simulink model "attitudeControllerSim"  (R2015b)
settings: Solver=VariableStepAuto  StartTime=0.0  StopTime=2  RelTol=1e-3
values from neighbouring files (symbols this model uses):
  pitch_ref = 0    [xyzController.m]
  roll_ref = 1    [xyzController.m]
undefined symbols (not defined in the file or in its folder): A12, Fg, Jx, Jy, Jz, kd, kth, L, Lobs, m, w1_bar, w2_bar, w3_bar, w4_bar
settings Model: Creator=USUARIO  LastModifiedBy=USUARIO

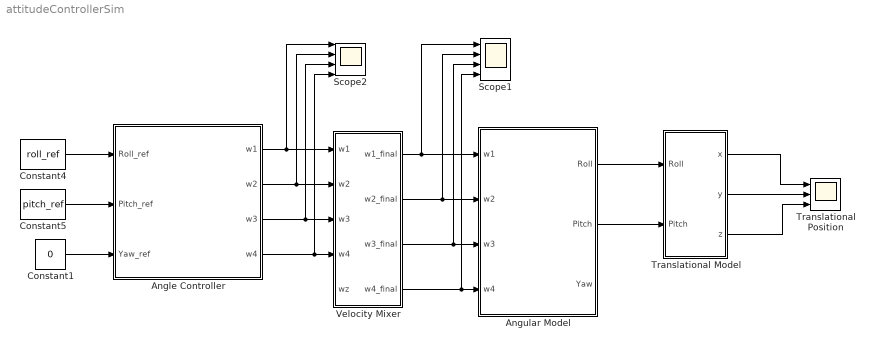
== system attitudeControllerSim ==
  Angle Controller : Subsystem
  Angular Model : Subsystem
  Constant1 : Constant  Value=0
  Constant4 : Constant  Value=roll_ref
  Constant5 : Constant  Value=pitch_ref
  Scope1 : Scope  NumInputPorts=4
  Scope2 : Scope  NumInputPorts=4
  Translational Position : Scope  NumInputPorts=3
  Translational Model : Subsystem
  Velocity Mixer : Subsystem
  wires:
  Constant1/1 -> Angle Controller/3(Yaw_ref)
  Velocity Mixer/1(w1_final) -> Scope1/1, Angular Model/1(w1)
  Velocity Mixer/2(w2_final) -> Scope1/2, Angular Model/2(w2)
  Velocity Mixer/3(w3_final) -> Scope1/3, Angular Model/3(w3)
  Velocity Mixer/4(w4_final) -> Scope1/4, Angular Model/4(w4)
  Angle Controller/1(w1) -> Velocity Mixer/1(w1), Scope2/1
  Angle Controller/2(w2) -> Velocity Mixer/2(w2), Scope2/2
  Angle Controller/3(w3) -> Velocity Mixer/3(w3), Scope2/3
  Angle Controller/4(w4) -> Velocity Mixer/4(w4), Scope2/4
  Angular Model/1(Roll) -> Translational Model/1(Roll)
  Translational Model/1(x) -> Translational Position/1
  Translational Model/2(y) -> Translational Position/2
  Translational Model/3(z) -> Translational Position/3
  Angular Model/2(Pitch) -> Translational Model/2(Pitch)
  Constant4/1 -> Angle Controller/1(Roll_ref)
  Constant5/1 -> Angle Controller/2(Pitch_ref)

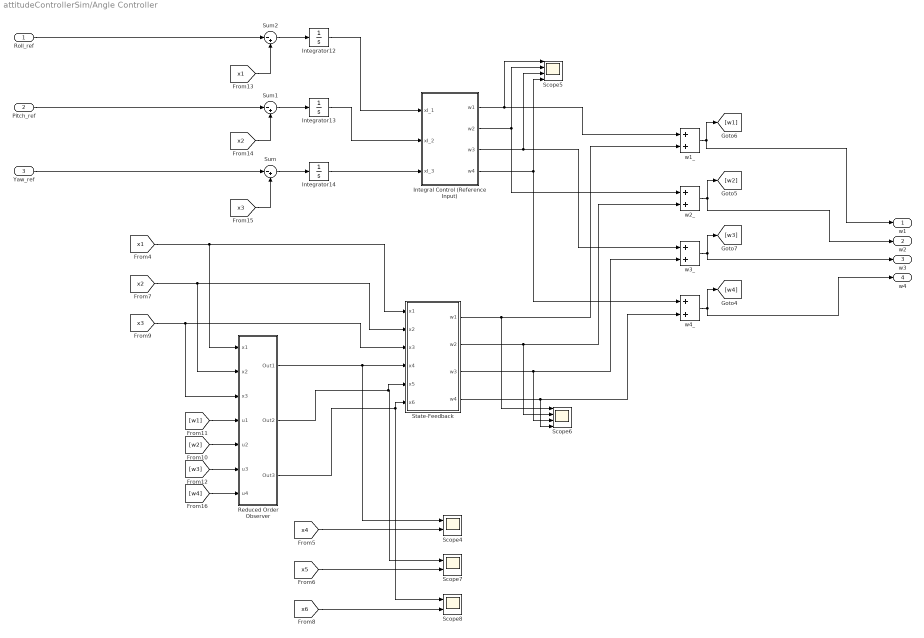
== system attitudeControllerSim/Angle Controller ==
  Roll_ref : Inport
  Pitch_ref : Inport  Port=2
  Yaw_ref : Inport  Port=3
  Integral Control (Reference Input) : MATLAB Function  TreatAsAtomicUnit=on
  Integrator12 : Integrator
  Integrator13 : Integrator
  Integrator14 : Integrator
  Reduced Order Observer : Subsystem
  Scope4 : Scope  NumInputPorts=2
  Scope5 : Scope  NumInputPorts=4
  Scope6 : Scope  NumInputPorts=4
  Scope7 : Scope  NumInputPorts=2
  Scope8 : Scope  NumInputPorts=2
  "State-Feedback " : MATLAB Function  TreatAsAtomicUnit=on
  Sum : Sum  Inputs=|-+
  Sum1 : Sum  Inputs=|-+
  Sum2 : Sum  Inputs=|-+
  w1_ : Sum
  w2_ : Sum
  w3_ : Sum
  w4_ : Sum
  w1 : Outport
  w2 : Outport  Port=2
  w3 : Outport  Port=3
  w4 : Outport  Port=4
  wires:
  "State-Feedback "/4(w4) -> w4_/2, Scope6/4
  Roll_ref/1 -> Sum2/1
  [x3] -> Sum/2
  [x1] -> Sum2/2
  Integrator13/1 -> Integral Control (Reference Input)/2(xI_2)
  "State-Feedback "/1(w1) -> w1_/2, Scope6/1
  [w3] -> Reduced Order Observer/6(u3)
  Sum2/1 -> Integrator12/1
  Sum/1 -> Integrator14/1
  [x3] -> "State-Feedback "/3(x3), Reduced Order Observer/3(x3)
  [w2] -> Reduced Order Observer/5(u2)
  Pitch_ref/1 -> Sum1/1
  Integrator14/1 -> Integral Control (Reference Input)/3(xI_3)
  Reduced Order Observer/3(Out3) -> "State-Feedback "/6(x6), Scope8/1
  [x4] -> Scope4/2
  [x6] -> Scope8/2
  "State-Feedback "/2(w2) -> w2_/2, Scope6/2
  Integral Control (Reference Input)/2(w2) -> Scope5/2, w2_/1
  [w4] -> Reduced Order Observer/7(u4)
  Integral Control (Reference Input)/3(w3) -> w3_/1, Scope5/3
  Reduced Order Observer/2(Out2) -> "State-Feedback "/5(x5), Scope7/1
  [x1] -> "State-Feedback "/1(x1), Reduced Order Observer/1(x1)
  [w1] -> Reduced Order Observer/4(u1)
  Integrator12/1 -> Integral Control (Reference Input)/1(xI_1)
  [x2] -> Sum1/2
  Integral Control (Reference Input)/4(w4) -> Scope5/4, w4_/1
  Integral Control (Reference Input)/1(w1) -> w1_/1, Scope5/1
  [x2] -> "State-Feedback "/2(x2), Reduced Order Observer/2(x2)
  Reduced Order Observer/1(Out1) -> "State-Feedback "/4(x4), Scope4/1
  [x5] -> Scope7/2
  Sum1/1 -> Integrator13/1
  Yaw_ref/1 -> Sum/1
  "State-Feedback "/3(w3) -> w3_/2, Scope6/3
  w1_/1 -> w1/1, [w1]
  w4_/1 -> w4/1, [w4]
  w2_/1 -> w2/1, [w2]
  w3_/1 -> w3/1, [w3]

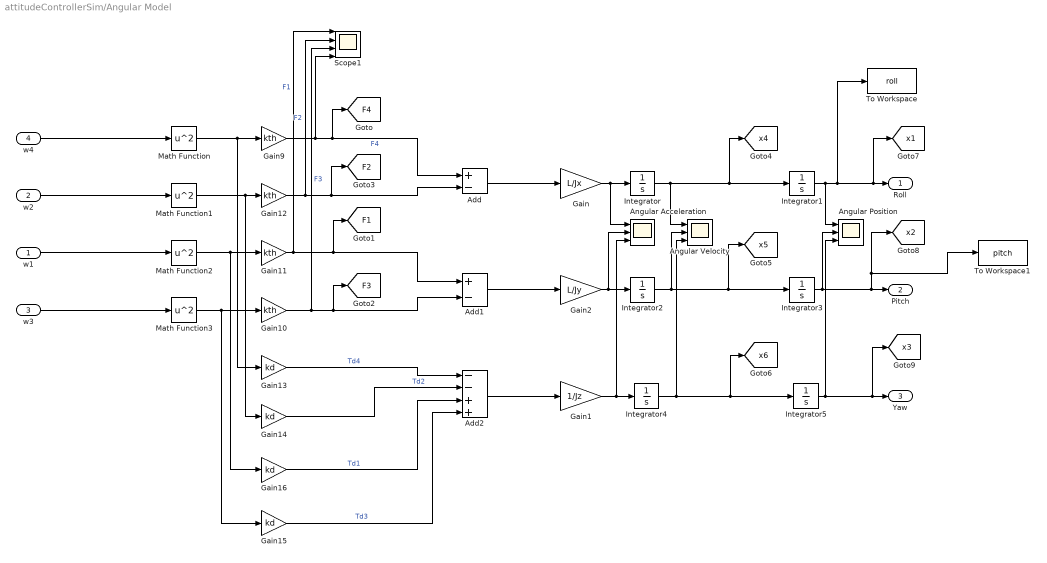
== system attitudeControllerSim/Angular Model ==
  w1 : Inport
  w2 : Inport  Port=2
  w3 : Inport  Port=3
  w4 : Inport  Port=4
  Add : Sum  Inputs=+-
  Add1 : Sum  Inputs=+-
  Add2 : Sum  Inputs=--++
  Angular Position : Scope  NumInputPorts=3
  Angular Velocity : Scope  NumInputPorts=3
  Angular Acceleration : Scope  NumInputPorts=3
  Gain : Gain  Gain=L/Jx
  Gain1 : Gain  Gain=1/Jz
  Gain{9..12} (4 alike) : Gain  Gain=kth
  Gain{13..16} (4 alike) : Gain  Gain=kd
  Gain2 : Gain  Gain=L/Jy
  Integrator{,1..5} (6 alike) : Integrator
  Math Function{,1..3} (4 alike) : Math  Operator=square  SaturateOnIntegerOverflow=on
  Scope1 : Scope  NumInputPorts=4
  To Workspace : ToWorkspace  VariableName=roll  SaveFormat=Timeseries  SampleTime=-1
  To Workspace1 : ToWorkspace  VariableName=pitch  SaveFormat=Timeseries  SampleTime=-1
  Roll : Outport
  Pitch : Outport  Port=2
  Yaw : Outport  Port=3
  tag scope: F1=global, F2=global, F3=global, F4=global, x1=global, x2=global, x3=global, x4=global, x5=global, x6=global
  wires:
  Gain2/1 -> Angular Acceleration/2, Integrator2/1
  Add2/1 -> Gain1/1
  Gain9/1 -> Scope1/4, [F4], Add/1  "F4"
  Gain14/1 -> Add2/2  "Td2"
  Gain16/1 -> Add2/3  "Td1"
  Gain/1 -> Angular Acceleration/1, Integrator/1
  Integrator/1 -> Angular Velocity/1, Integrator1/1, [x4]
  Integrator1/1 -> To Workspace/1, [x1], Roll/1, Angular Position/1
  Integrator4/1 -> Angular Velocity/3, [x6], Integrator5/1
  Add/1 -> Gain/1
  Integrator3/1 -> To Workspace1/1, [x2], Pitch/1, Angular Position/2
  Add1/1 -> Gain2/1
  Integrator5/1 -> Angular Position/3, [x3], Yaw/1
  Gain12/1 -> Scope1/2, [F2], Add/2  "F2"
  Gain10/1 -> [F3], Add1/2, Scope1/3  "F3"
  Gain11/1 -> Scope1/1, [F1], Add1/1  "F1"
  Gain13/1 -> Add2/1  "Td4"
  Gain15/1 -> Add2/4  "Td3"
  Integrator2/1 -> Angular Velocity/2, [x5], Integrator3/1
  Gain1/1 -> Angular Acceleration/3, Integrator4/1
  Math Function3/1 -> Gain15/1, Gain10/1
  Math Function2/1 -> Gain16/1, Gain11/1
  Math Function/1 -> Gain13/1, Gain9/1
  Math Function1/1 -> Gain14/1, Gain12/1
  w1/1 -> Math Function2/1
  w2/1 -> Math Function1/1
  w3/1 -> Math Function3/1
  w4/1 -> Math Function/1

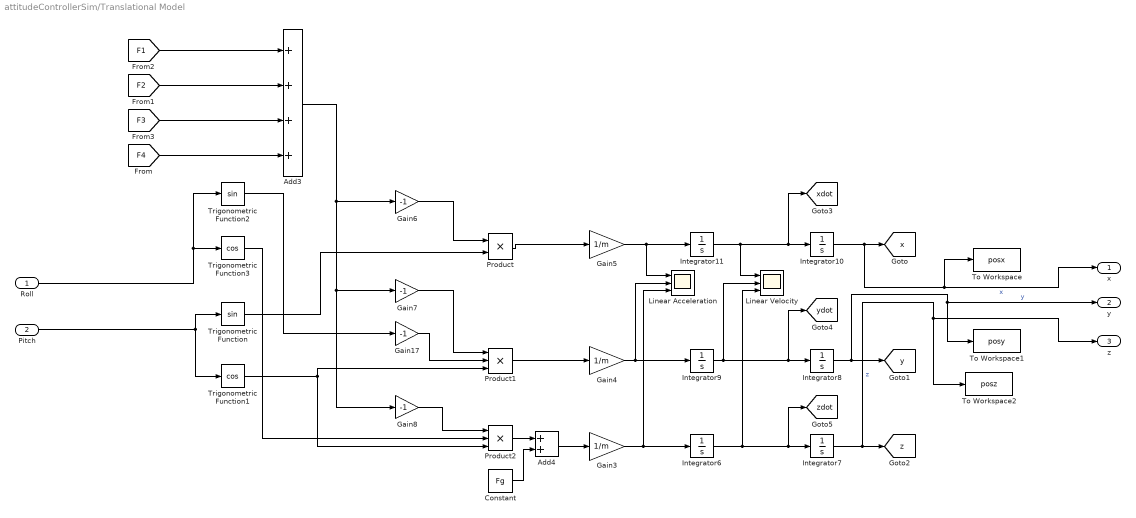
== system attitudeControllerSim/Translational Model ==
  Roll : Inport
  Pitch : Inport  Port=2
  Add3 : Sum  Inputs=4
  Add4 : Sum  Inputs=2
  Constant : Constant  Value=Fg
  Gain{6..8,17} (4 alike) : Gain  Gain=-1
  Gain3 : Gain  Gain=1/m
  Gain4 : Gain  Gain=1/m
  Gain5 : Gain  Gain=1/m
  Integrator{6..11} (6 alike) : Integrator
  Linear Acceleration : Scope  NumInputPorts=3
  Linear Velocity : Scope  NumInputPorts=3
  Product : Product
  Product1 : Product  Inputs=3
  Product2 : Product  Inputs=3
  To Workspace : ToWorkspace  VariableName=posx  SampleTime=-1
  To Workspace1 : ToWorkspace  VariableName=posy  SampleTime=-1
  To Workspace2 : ToWorkspace  VariableName=posz  SampleTime=-1
  Trigonometric Function : Trigonometry
  Trigonometric Function1 : Trigonometry  Operator=cos
  Trigonometric Function2 : Trigonometry
  Trigonometric Function3 : Trigonometry  Operator=cos
  x : Outport
  y : Outport  Port=2
  z : Outport  Port=3
  tag scope: x=global, xdot=global, y=global, ydot=global, z=global, zdot=global
  wires:
  Product/1 -> Gain5/1
  Product1/1 -> Gain4/1
  Gain4/1 -> Integrator9/1, Linear Acceleration/2
  Gain5/1 -> Integrator11/1, Linear Acceleration/1
  Add4/1 -> Gain3/1
  Roll/1 -> Trigonometric Function2/1, Trigonometric Function3/1
  Trigonometric Function3/1 -> Product2/2
  Integrator10/1 -> [x], x/1, To Workspace/1  "x"
  Add3/1 -> Gain8/1, Gain7/1, Gain6/1
  Gain8/1 -> Product2/1
  [F2] -> Add3/2
  [F4] -> Add3/4
  Trigonometric Function/1 -> Product/2
  Integrator7/1 -> z/1, To Workspace2/1, [z]  "z"
  [F1] -> Add3/1
  Product2/1 -> Add4/1
  Trigonometric Function2/1 -> Gain17/1
  Integrator6/1 -> [zdot], Integrator7/1, Linear Velocity/3
  Gain17/1 -> Product1/2
  Constant/1 -> Add4/2
  Trigonometric Function1/1 -> Product2/3, Product1/3
  Integrator9/1 -> [ydot], Integrator8/1, Linear Velocity/2
  Integrator8/1 -> y/1, To Workspace1/1, [y]  "y"
  Gain6/1 -> Product/1
  Gain7/1 -> Product1/1
  [F3] -> Add3/3
  Pitch/1 -> Trigonometric Function/1, Trigonometric Function1/1
  Integrator11/1 -> [xdot], Integrator10/1, Linear Velocity/1
  Gain3/1 -> Integrator6/1, Linear Acceleration/3

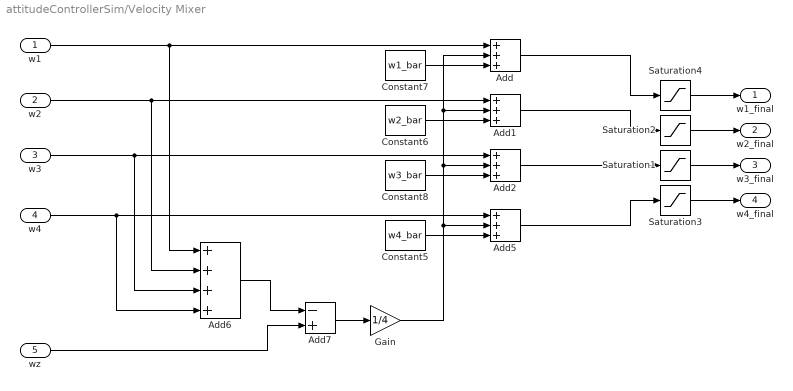
== system attitudeControllerSim/Velocity Mixer ==
  w1 : Inport
  w2 : Inport  Port=2
  w3 : Inport  Port=3
  w4 : Inport  Port=4
  wz : Inport  Port=5
  Add{,1..2,5} (4 alike) : Sum  Inputs=+++
  Add6 : Sum  Inputs=4
  Add7 : Sum  Inputs=-+
  Constant5 : Constant  Value=w4_bar
  Constant6 : Constant  Value=w2_bar
  Constant7 : Constant  Value=w1_bar
  Constant8 : Constant  Value=w3_bar
  Gain : Gain  Gain=1/4
  Saturation{1..4} (4 alike) : Saturate  UpperLimit=500  LowerLimit=300
  w1_final : Outport
  w2_final : Outport  Port=2
  w3_final : Outport  Port=3
  w4_final : Outport  Port=4
  wires:
  w4/1 -> Add6/4, Add5/1
  Gain/1 -> Add1/2, Add/2, Add2/2, Add5/2
  Add7/1 -> Gain/1
  Add6/1 -> Add7/1
  w2/1 -> Add6/2, Add1/1
  w3/1 -> Add6/3, Add2/1
  wz/1 -> Add7/2
  Add/1 -> Saturation4/1
  Add1/1 -> Saturation2/1
  Add2/1 -> Saturation1/1
  Add5/1 -> Saturation3/1
  w1/1 -> Add/1, Add6/1
  Constant7/1 -> Add/3
  Constant6/1 -> Add1/3
  Constant8/1 -> Add2/3
  Constant5/1 -> Add5/3
  Saturation2/1 -> w2_final/1
  Saturation1/1 -> w3_final/1
  Saturation4/1 -> w1_final/1
  Saturation3/1 -> w4_final/1

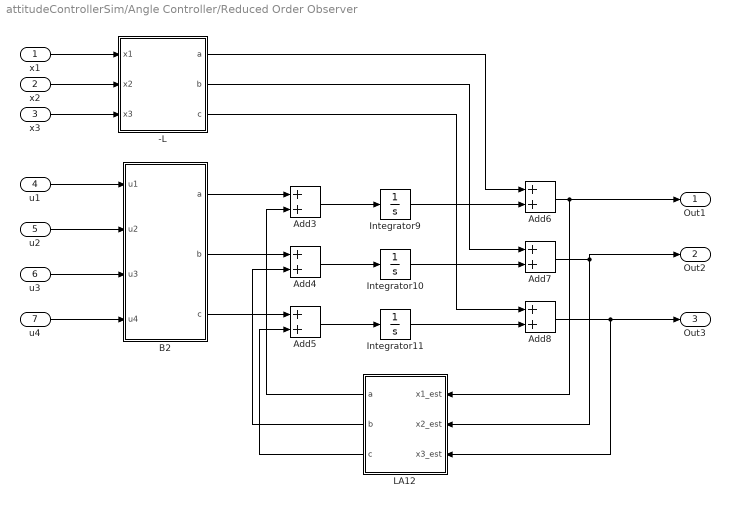
== system attitudeControllerSim/Angle Controller/Reduced Order Observer ==
  x1 : Inport
  x2 : Inport  Port=2
  x3 : Inport  Port=3
  u1 : Inport  Port=4
  u2 : Inport  Port=5
  u3 : Inport  Port=6
  u4 : Inport  Port=7
  "-L " : MATLAB Function  TreatAsAtomicUnit=on
  Add{3..8} (6 alike) : Sum  Inputs=2
  B2 : MATLAB Function  TreatAsAtomicUnit=on
  Integrator10 : Integrator
  Integrator11 : Integrator
  Integrator9 : Integrator
  LA12 : MATLAB Function  TreatAsAtomicUnit=on
  Out1 : Outport
  Out2 : Outport  Port=2
  Out3 : Outport  Port=3
  wires:
  Add4/1 -> Integrator10/1
  Add3/1 -> Integrator9/1
  Add5/1 -> Integrator11/1
  u4/1 -> B2/4(u4)
  u2/1 -> B2/2(u2)
  B2/1(a) -> Add3/1
  B2/2(b) -> Add4/1
  B2/3(c) -> Add5/1
  LA12/1(a) -> Add3/2
  LA12/2(b) -> Add4/2
  LA12/3(c) -> Add5/2
  Add6/1 -> LA12/1(x1_est), Out1/1
  Add7/1 -> LA12/2(x2_est), Out2/1
  Add8/1 -> LA12/3(x3_est), Out3/1
  "-L "/3(c) -> Add8/1
  "-L "/1(a) -> Add6/1
  "-L "/2(b) -> Add7/1
  x2/1 -> "-L "/2(x2)
  x3/1 -> "-L "/3(x3)
  x1/1 -> "-L "/1(x1)
  Integrator9/1 -> Add6/2
  Integrator11/1 -> Add8/2
  Integrator10/1 -> Add7/2
  u1/1 -> B2/1(u1)
  u3/1 -> B2/3(u3)

== matlab function attitudeControllerSim/Angle Controller/State-Feedback  ==
  data: x1 input; w1 output; w2 output; w3 output; w4 output; x2 input; x3 input; x4 input; x5 input; x6 input; F parameter
function [w1,w2,w3,w4] = F_matrix(x1, x2, x3, x4, x5, x6, F)
x=[x1;
    x2;
    x3;
    x4;
    x5;
    x6];

w=F*x;

w1=w(1);
w2=w(2);
w3=w(3);
w4=w(4);

== matlab function attitudeControllerSim/Angle Controller/Integral Control (Reference Input) ==
  data: xI_1 input; w1 output; w2 output; w3 output; w4 output; xI_2 input; xI_3 input; FI parameter
function [w1,w2,w3,w4] = FI_matrix(xI_1, xI_2, xI_3,FI)
xI=[xI_1;
    xI_2;
    xI_3];

w=FI*xI;

w1=w(1);
w2=w(2);
w3=w(3);
w4=w(4);

== matlab function attitudeControllerSim/Angle Controller/Reduced Order Observer/-L  ==
  data: x1 input; a output; b output; c output; x2 input; x3 input; Lobs parameter
function [a,b,c] = minusL_matrix(x1, x2, x3, Lobs)
x=[x1;
    x2;
    x3];

abc=-Lobs*x;

a=abc(1);
b=abc(2);
c=abc(3);

== matlab function attitudeControllerSim/Angle Controller/Reduced Order Observer/B2 ==
  data: u1 input; a output; b output; c output; u2 input; u3 input; u4 input; B2 parameter
function [a, b, c] = B2_matrix(u1, u2, u3, u4, B2)
u=[u1;
    u2;
    u3;
    u4];

abc=B2*u;

a=abc(1);
b=abc(2);
c=abc(3);

== matlab function attitudeControllerSim/Angle Controller/Reduced Order Observer/LA12 ==
  data: x1_est input; x2_est input; x3_est input; a output; b output; c output; Lobs parameter; A12 parameter
function [a,b,c] = LA12_matrix(x1_est, x2_est, x3_est, Lobs, A12)
x=[x1_est;
    x2_est;
    x3_est];

abc=Lobs*A12*x;

a=abc(1);
b=abc(2);
c=abc(3);
